simulink model "model"  (R2025b)
settings: Solver=VariableStepAuto  StartTime=0.0  StopTime=50  RelTol=1e-3
values from neighbouring files (symbols this model uses):
  A = [0 1; -2 -3]    [init.m]
  A0 = [0  1 ... (first row only)    [init.m]
  B = [0; 9]    [init.m]
  C = [1 0]    [init.m]
  e_U = [0;1]    [init.m]
  e_Y0 = [0;1]    [init.m]
  e_Y1 = [1;0]    [init.m]
  gamma = 1    [init.m]
  I = eye(2)    [init.m]
  v0 = [0;0]    [init.m]
  x0 = [0;0]    [init.m]
settings Model: Creator=eva  LastModifiedBy=eva

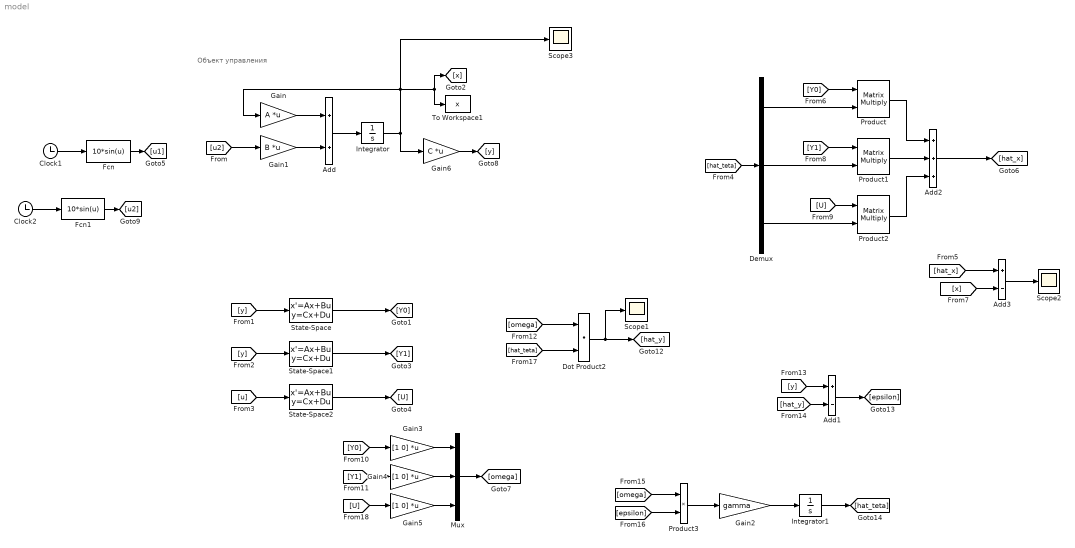
== system model ==
  note: Объект управления
  Add : Sum
  Add1 : Sum  Inputs=+-
  Add2 : Sum  Inputs=+++
  Add3 : Sum  Inputs=+-
  Clock1 : Clock
  Clock2 : Clock
  Demux : Demux  Outputs=3
  Dot Product2 : DotProduct  OutDataTypeStr=Inherit: Inherit via internal rule
  Fcn : Fcn  Expr=10*sin(u)
  Fcn1 : Fcn  Expr=10*sin(u)
  Gain : Gain  Gain=A  Multiplication=Matrix(K*u)
  Gain1 : Gain  Gain=B  Multiplication=Matrix(K*u)
  Gain2 : Gain  Gain=gamma
  Gain3 : Gain  Gain=[1 0]  Multiplication=Matrix(K*u)
  Gain4 : Gain  Gain=[1 0]  Multiplication=Matrix(K*u)
  Gain5 : Gain  Gain=[1 0]  Multiplication=Matrix(K*u)
  Gain6 : Gain  Gain=C  Multiplication=Matrix(K*u)
  Integrator : Integrator  InitialCondition=[0; 0]
  Integrator1 : Integrator  InitialCondition=[0;0;0]
  Mux : Mux  Inputs=3
  Product : Product  Multiplication=Matrix(*)
  Product1 : Product  Multiplication=Matrix(*)
  Product2 : Product  Multiplication=Matrix(*)
  Product3 : Product
  Scope1 : Scope
      settings: ActiveDisplayYMinimum=-1  ActiveDisplayYMaximum=1
  Scope2 : Scope
      settings: ActiveDisplayYMinimum=-112.97863638113148  ActiveDisplayYMaximum=50.937899091779464
  Scope3 : Scope
      settings: ActiveDisplayYMinimum=-1  ActiveDisplayYMaximum=1  DataLoggingVariableName=ScopeData2
  State-Space : StateSpace  A=A0  B=e_Y0  C=I  D=v0  InitialCondition=x0
  State-Space1 : StateSpace  A=A0  B=e_Y1  C=I  D=v0  InitialCondition=x0
  State-Space2 : StateSpace  A=A0  B=e_U  C=I  D=v0  InitialCondition=x0
  To Workspace1 : ToWorkspace  VariableName=x  SaveFormat=Structure With Time  SampleTime=-1
  wires:
  [u2] -> Gain1/1
  Gain/1 -> Add/1
  Add/1 -> Integrator/1
  Gain1/1 -> Add/2
  Integrator/1 -> Gain6/1, Scope3/1, To Workspace1/1, [x], Gain/1
  Gain6/1 -> [y]
  [y] -> State-Space/1
  State-Space/1 -> [Y0]
  State-Space1/1 -> [Y1]
  [y] -> State-Space1/1
  [u] -> State-Space2/1
  State-Space2/1 -> [U]
  [omega] -> Dot Product2/1
  [hat_teta] -> Dot Product2/2
  Dot Product2/1 -> Scope1/1, [hat_y]
  [y] -> Add1/1
  [hat_y] -> Add1/2
  Add1/1 -> [epsilon]
  Product3/1 -> Gain2/1
  [epsilon] -> Product3/2
  [omega] -> Product3/1
  Gain2/1 -> Integrator1/1
  Integrator1/1 -> [hat_teta]
  Clock1/1 -> Fcn/1
  Fcn/1 -> [u1]
  [hat_teta] -> Demux/1
  [Y0] -> Product/1
  Demux/1 -> Product/2
  Demux/2 -> Product1/2
  [Y1] -> Product1/1
  [U] -> Product2/1
  Product/1 -> Add2/1
  Product1/1 -> Add2/2
  Product2/1 -> Add2/3
  Demux/3 -> Product2/2
  Add2/1 -> [hat_x]
  Gain4/1 -> Mux/2
  Gain3/1 -> Mux/1
  Mux/1 -> [omega]
  Gain5/1 -> Mux/3
  [hat_x] -> Add3/1
  [x] -> Add3/2
  [Y0] -> Gain3/1
  [Y1] -> Gain4/1
  [U] -> Gain5/1
  Add3/1 -> Scope2/1
  Fcn1/1 -> [u2]
  Clock2/1 -> Fcn1/1
